simulink model "Symmetry_Inverter"  (Simulink 8.3)
settings: Solver=ode23t  StartTime=0.0  StopTime=tfin  RelTol=1e-4
values from neighbouring files (symbols this model uses):
  amp_feedback_saturation = 400    [Symmetry_ini_COPY.m]
  Bridge_Inductances = 4e-3    (= 0.004)    [Inverter_ini.m]    (also in Symmetry_ini_COPY.m)
  Buffer_Capacitance = 10e-3    (= 0.01)    [Inverter_ini.m]    (also in Symmetry_ini_COPY.m)
  C_Network = [0, 0, 0]    [Symmetry_ini.m]    (also in Symmetry_ini_COPY.m)
  Capacitive_Load_R_RC = [30e-3,  60e-3,  40e-3;                                1e-3, 5e-3, 3e-3]    [Symmetry_ini.m]    (also in Symmetry_ini_COPY.m = [60e-3,  120e-3,  80e-3;                                 1e-)
  Capacitive_Load_S_RC = [30e-3,  60e-3,  40e-3;                                1e-3, 5e-3, 3e-3]    [Symmetry_ini.m]    (also in Symmetry_ini_COPY.m = [60e-3,  120e-3,  80e-3;                                1e-3)
  Capacitive_Load_T_RC = [30e-3,  60e-3,  40e-3;                                1e-3, 5e-3, 3e-3]    [Symmetry_ini.m]    (also in Symmetry_ini_COPY.m = [60e-3,  120e-3,  80e-3;                                 1e-)
  i = str2num(answer{1})/sample    [Test_intersect.m]
  initial_value = [0.00,0.00,0.00,                  0,0,0]    [Symmetry_ini_COPY.m]
  L_Network = [3.185e-3, 3.185e-3, 3.185e-3, 3.185e-3]    [Symmetry_ini.m]    (also in Symmetry_ini_COPY.m)
  L_Source = [3.185e-3, 3.185e-3, 3.185e-3]    [Sketch_controller_model_ini.m]    (also in Symmetry_ini.m; Symmetry_ini_COPY.m)
  Load_R = [50,50,50]    [Symmetry_ini.m]    (also in Symmetry_ini_COPY.m)
  Load_RL = [35.35,   35.35,   35.35;                  0.1125,  0.1125,  0.1125]    [Symmetry_ini.m]    (also in Symmetry_ini_COPY.m = [35.35,   35.35,   35.35;                   0.1125,  0.1125,)
  Load_Wire_Resistance = [0.1,0.2]    [Symmetry_ini.m]    (also in Symmetry_ini_COPY.m)
  P_gain = 0.00001    (= 1e-05)    [Symmetry_ini_COPY.m]
  phase_feedback_saturation = pi    (= 3.14159265359)    [Symmetry_ini_COPY.m]
  Phase_Source = [0,2/3*pi,4/3*pi]    [Sketch_controller_model_ini.m]    (also in Symmetry_REAL_TIME_ini.m = [0,-2/3*pi,-4/3*pi]; Symmetry_ini.m; Symmetry_ini_COPY.m = [0,-2/3*pi,-4/3*pi])
  R_Network = [0.4, 0.4, 0.4, 0.4]    [Symmetry_ini.m]    (also in Symmetry_ini_COPY.m)
  R_Source = [0.4, 0.4, 0.4]    [Sketch_controller_model_ini.m]    (also in Symmetry_ini.m; Symmetry_ini_COPY.m)
  sample = 10e-5    (= 0.0001)    [Inverter_ini.m]    (also in Sketch_controller_model_ini.m; Symmetry_REAL_TIME_ini.m; Symmetry_ini.m; Symmetry_ini_COPY.m)
  Source_Frequency = [50,50,50]    [Sketch_controller_model_ini.m]    (also in Symmetry_ini.m; Symmetry_ini_COPY.m)
  Start_Control = 1    [Symmetry_ini_COPY.m]
  START_Load_R = [0.001,100,100]    [Symmetry_ini_COPY.m]
  START_Load_RC = [100,100,0.001]    [Symmetry_ini_COPY.m]
  START_Load_RL = [100,0.001,100]    [Symmetry_ini_COPY.m]
  step_size = [5,5,5,                  0.36,0.36,0.36]    [Symmetry_ini_COPY.m]
  test_step = [0.5,0.5,0.5,                  0.02,0.02,0.02]    [Symmetry_ini_COPY.m]
  Urms_Source = [230,230,230]    [Sketch_controller_model_ini.m]    (also in Symmetry_REAL_TIME_ini.m; Symmetry_ini.m; Symmetry_ini_COPY.m)
undefined symbols (not defined in the file or in its folder): Ion, Lithium
libraries: powerlib x132, simulink x23, dspsigops x14, commsequence2 x6, dspxfrm3 x3, dsparch4 x2, electricdrivelib x1
(part 2 of 2)

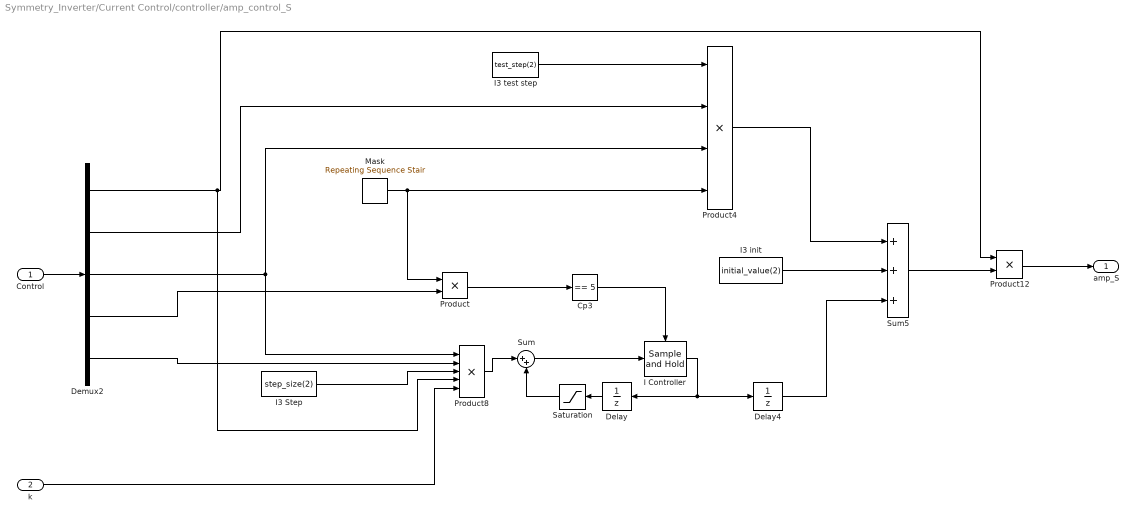
== system Symmetry_Inverter/Current Control/controller/amp_control_S ==
  Control : Inport
  k : Inport  Port=2
  Cp3 : simulink/Logic and Bit Operations/Compare To Constant  relop===  const=5  OutDataTypeStr=uint8  ZeroCross=off
  Delay : UnitDelay  SampleTime=0.001
  Delay4 : UnitDelay  SampleTime=0.02
  Demux2 : Demux  Outputs=5
  I Controller : dspsigops/Sample and Hold  trig=Rising edge  initCond=0  latchinput=off
  I3 Step : Constant  Value=step_size(2)
  "I3 init " : Constant  Value=initial_value(2)
  I3 test step : Constant  Value=test_step(2)
  Mask : simulink/Sources/Repeating Sequence Stair  OutValues=[0 1 0 0 0 0].'  tsamp=mask_sample  OutMin=[]  OutMax=[]  OutDataTypeStr=float('double')  OutputDataTypeScalingMode=Specify via dialog  OutDataType=float('double')  ConRadixGroup=Best Precision: Vector-wise  OutScaling=2^-12
  Product : Product  RndMeth=Zero
  Product12 : Product  RndMeth=Zero
  Product4 : Product  Inputs=4  RndMeth=Zero
  Product8 : Product  Inputs=5  RndMeth=Zero
  Saturation : Saturate  UpperLimit=amp_feedback_saturation  LowerLimit=-amp_feedback_saturation
  Sum : Sum  Inputs=|++
  Sum5 : Sum  Inputs=+++
  amp_S : Outport
  wires:
  Saturation/1 -> Sum/2
  Sum/1 -> I Controller/1
  Product/1 -> Cp3/1
  Product4/1 -> Sum5/1
  I Controller/1 -> Delay/1, Delay4/1
  I3 test step/1 -> Product4/1
  Sum5/1 -> Product12/2
  Mask/1 -> Product4/4, Product/1
  Cp3/1 -> I Controller/Trigger
  I3 Step/1 -> Product8/3
  Demux2/1 -> Product8/4, Product12/1
  Demux2/2 -> Product4/2
  Demux2/3 -> Product8/1, Product4/3
  Demux2/4 -> Product/2
  Demux2/5 -> Product8/2
  Delay4/1 -> Sum5/3
  "I3 init "/1 -> Sum5/2
  Delay/1 -> Saturation/1
  Product8/1 -> Sum/1
  Product12/1 -> amp_S/1
  Control/1 -> Demux2/1
  k/1 -> Product8/5

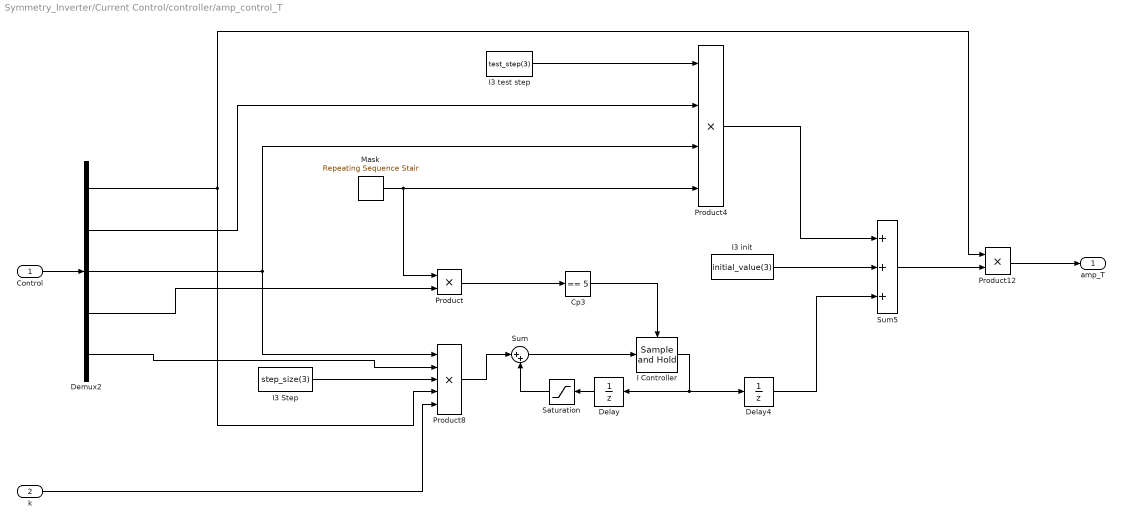
== system Symmetry_Inverter/Current Control/controller/amp_control_T ==
  Control : Inport
  k : Inport  Port=2
  Cp3 : simulink/Logic and Bit Operations/Compare To Constant  relop===  const=5  OutDataTypeStr=uint8  ZeroCross=off
  Delay : UnitDelay  SampleTime=0.001
  Delay4 : UnitDelay  SampleTime=0.02
  Demux2 : Demux  Outputs=5
  I Controller : dspsigops/Sample and Hold  trig=Rising edge  initCond=0  latchinput=off
  I3 Step : Constant  Value=step_size(3)
  "I3 init " : Constant  Value=initial_value(3)
  I3 test step : Constant  Value=test_step(3)
  Mask : simulink/Sources/Repeating Sequence Stair  OutValues=[0 0 1 0 0 0].'  tsamp=mask_sample  OutMin=[]  OutMax=[]  OutDataTypeStr=float('double')  OutputDataTypeScalingMode=Specify via dialog  OutDataType=float('double')  ConRadixGroup=Best Precision: Vector-wise  OutScaling=2^-12
  Product : Product  RndMeth=Zero
  Product12 : Product  RndMeth=Zero
  Product4 : Product  Inputs=4  RndMeth=Zero
  Product8 : Product  Inputs=5  RndMeth=Zero
  Saturation : Saturate  UpperLimit=amp_feedback_saturation  LowerLimit=-amp_feedback_saturation
  Sum : Sum  Inputs=|++
  Sum5 : Sum  Inputs=+++
  amp_T : Outport
  wires:
  Control/1 -> Demux2/1
  Product12/1 -> amp_T/1
  Product8/1 -> Sum/1
  Delay/1 -> Saturation/1
  "I3 init "/1 -> Sum5/2
  Delay4/1 -> Sum5/3
  Demux2/5 -> Product8/2
  Demux2/4 -> Product/2
  Demux2/3 -> Product4/3, Product8/1
  Demux2/2 -> Product4/2
  Demux2/1 -> Product12/1, Product8/4
  I3 Step/1 -> Product8/3
  Cp3/1 -> I Controller/Trigger
  Mask/1 -> Product/1, Product4/4
  Sum5/1 -> Product12/2
  I3 test step/1 -> Product4/1
  I Controller/1 -> Delay4/1, Delay/1
  Product4/1 -> Sum5/1
  Product/1 -> Cp3/1
  Sum/1 -> I Controller/1
  Saturation/1 -> Sum/2
  k/1 -> Product8/5

== system Symmetry_Inverter/Current Control/controller/phase_control_R ==
  Control : Inport
  Cp3 : simulink/Logic and Bit Operations/Compare To Constant  relop===  const=5  OutDataTypeStr=uint8  ZeroCross=off
  Delay : UnitDelay  SampleTime=0.001
  Delay4 : UnitDelay  SampleTime=0.02
  Demux2 : Demux  Outputs=5
  I Controller : dspsigops/Sample and Hold  trig=Rising edge  initCond=0  latchinput=off
  I3 Step : Constant  Value=step_size(4)
  "I3 init " : Constant  Value=initial_value(4)
  I3 test step : Constant  Value=test_step(4)
  Mask : simulink/Sources/Repeating Sequence Stair  OutValues=[0 0 0 1 0 0].'  tsamp=mask_sample  OutMin=[]  OutMax=[]  OutDataTypeStr=float('double')  OutputDataTypeScalingMode=Specify via dialog  OutDataType=float('double')  ConRadixGroup=Best Precision: Vector-wise  OutScaling=2^-12
  Product : Product  RndMeth=Zero
  Product12 : Product  RndMeth=Zero
  Product4 : Product  Inputs=4  RndMeth=Zero
  Product8 : Product  Inputs=4  RndMeth=Zero
  Saturation : Saturate  UpperLimit=phase_feedback_saturation  LowerLimit=-phase_feedback_saturation
  Sum : Sum  Inputs=|++
  Sum5 : Sum  Inputs=+++
  phase_R : Outport
  wires:
  Saturation/1 -> Sum/2
  Sum/1 -> I Controller/1
  Product/1 -> Cp3/1
  Product4/1 -> Sum5/1
  I Controller/1 -> Delay/1, Delay4/1
  I3 test step/1 -> Product4/1
  Sum5/1 -> Product12/2
  Mask/1 -> Product4/4, Product/1
  Cp3/1 -> I Controller/Trigger
  I3 Step/1 -> Product8/3
  Demux2/1 -> Product12/1, Product8/4
  Demux2/2 -> Product4/2
  Demux2/3 -> Product8/1, Product4/3
  Demux2/4 -> Product/2
  Demux2/5 -> Product8/2
  Delay4/1 -> Sum5/3
  "I3 init "/1 -> Sum5/2
  Delay/1 -> Saturation/1
  Product8/1 -> Sum/1
  Product12/1 -> phase_R/1
  Control/1 -> Demux2/1

== system Symmetry_Inverter/Current Control/controller/phase_control_T ==
  Control : Inport
  Cp3 : simulink/Logic and Bit Operations/Compare To Constant  relop===  const=5  OutDataTypeStr=uint8  ZeroCross=off
  Delay : UnitDelay  SampleTime=0.001
  Delay4 : UnitDelay  SampleTime=0.02
  Demux2 : Demux  Outputs=5
  I Controller : dspsigops/Sample and Hold  trig=Rising edge  initCond=0  latchinput=off
  I3 Step : Constant  Value=step_size(6)
  "I3 init " : Constant  Value=initial_value(6)
  I3 test step : Constant  Value=test_step(6)
  Mask : simulink/Sources/Repeating Sequence Stair  OutValues=[0 0 0 0 0 1].'  tsamp=mask_sample  OutMin=[]  OutMax=[]  OutDataTypeStr=float('double')  OutputDataTypeScalingMode=Specify via dialog  OutDataType=float('double')  ConRadixGroup=Best Precision: Vector-wise  OutScaling=2^-12
  Product : Product  RndMeth=Zero
  Product12 : Product  RndMeth=Zero
  Product4 : Product  Inputs=4  RndMeth=Zero
  Product8 : Product  Inputs=4  RndMeth=Zero
  Saturation : Saturate  UpperLimit=phase_feedback_saturation  LowerLimit=-phase_feedback_saturation
  Sum : Sum  Inputs=|++
  Sum5 : Sum  Inputs=+++
  phase_S : Outport
  wires:
  Saturation/1 -> Sum/2
  Sum/1 -> I Controller/1
  Product/1 -> Cp3/1
  Product4/1 -> Sum5/1
  I Controller/1 -> Delay/1, Delay4/1
  I3 test step/1 -> Product4/1
  Sum5/1 -> Product12/2
  Mask/1 -> Product4/4, Product/1
  Cp3/1 -> I Controller/Trigger
  I3 Step/1 -> Product8/3
  Demux2/1 -> Product12/1, Product8/4
  Demux2/2 -> Product4/2
  Demux2/3 -> Product8/1, Product4/3
  Demux2/4 -> Product/2
  Demux2/5 -> Product8/2
  Delay4/1 -> Sum5/3
  "I3 init "/1 -> Sum5/2
  Delay/1 -> Saturation/1
  Product8/1 -> Sum/1
  Product12/1 -> phase_S/1
  Control/1 -> Demux2/1

== system Symmetry_Inverter/Load System/Loads/Capacitive_Loads_RST ==
  Breaker1 : powerlib/Elements/Breaker  InitialState=0  SwitchingTimes="[ 1/60  5/60 ]"  External=on  BreakerResistance=0.01  SnubberResistance=1e7  SnubberCapacitance=inf  Measurements=None  MoreParameters=off  NoBreakLoop=off
  Breaker4 : powerlib/Elements/Breaker  InitialState=0  SwitchingTimes="[ 1/60  5/60 ]"  External=on  BreakerResistance=0.01  SnubberResistance=1e7  SnubberCapacitance=inf  Measurements=None  MoreParameters=off  NoBreakLoop=off
  Breaker6 : powerlib/Elements/Breaker  InitialState=0  SwitchingTimes="[ 1/60  5/60 ]"  External=on  BreakerResistance=0.01  SnubberResistance=1e7  SnubberCapacitance=inf  Measurements=None  MoreParameters=off  NoBreakLoop=off
  Capacitive_Load_R : Subsystem
  Capacitive_Load_S : Subsystem
  Capacitive_Load_T : Subsystem
  Clock : Clock
      settings: Decimation=CLK
  const : Constant
  const1 : Constant  Value=0
  on/off : Switch  Criteria=u2 > Threshold  Threshold=START_Load_RC(1)
  on/off1 : Switch  Criteria=u2 > Threshold  Threshold=START_Load_RC(2)
  on/off2 : Switch  Criteria=u2 > Threshold  Threshold=START_Load_RC(3)
  R : PMIOPort  Port=1  Side=Right
  S : PMIOPort  Port=2  Side=Right
  T : PMIOPort  Port=3  Side=Right
  N : PMIOPort  Port=4  Side=Left
  wires:
  const/1 -> on/off2/1, on/off1/1, on/off/1
  const1/1 -> on/off2/3, on/off1/3, on/off/3
  Clock/1 -> on/off2/2, on/off1/2, on/off/2
  on/off/1 -> Breaker4/1
  on/off1/1 -> Breaker1/1
  on/off2/1 -> Breaker6/1
  connections:
  R/RConn1 -- Breaker4/LConn1
  S/RConn1 -- Breaker1/LConn1
  T/RConn1 -- Breaker6/LConn1
  Capacitive_Load_R/LConn1 -- Breaker4/RConn1
  Capacitive_Load_S/LConn1 -- Breaker1/RConn1
  Capacitive_Load_T/LConn1 -- Breaker6/RConn1
  Capacitive_Load_R/LConn2 -- Capacitive_Load_S/LConn2 -- Capacitive_Load_T/LConn2 -- N/RConn1

== system Symmetry_Inverter/Load System/Loads/Inductive_Loads_RST ==
  Breaker1 : powerlib/Elements/Breaker  InitialState=0  SwitchingTimes="[ 1/60  5/60 ]"  External=on  BreakerResistance=0.01  SnubberResistance=1e7  SnubberCapacitance=inf  Measurements=None  MoreParameters=off  NoBreakLoop=off
  Breaker13 : powerlib/Elements/Breaker  InitialState=0  SwitchingTimes="[ 1/60  5/60 ]"  External=on  BreakerResistance=0.01  SnubberResistance=1e7  SnubberCapacitance=inf  Measurements=None  MoreParameters=off  NoBreakLoop=off
  Breaker2 : powerlib/Elements/Breaker  InitialState=0  SwitchingTimes="[ 1/60  5/60 ]"  External=on  BreakerResistance=0.01  SnubberResistance=1e7  SnubberCapacitance=inf  Measurements=None  MoreParameters=off  NoBreakLoop=off
  Clock : Clock
      settings: Decimation=CLK
  RL_load : powerlib/Elements/Series RLC Branch  LConnTagsString=__new0  RConnTagsString=__new0  BranchType=RL  Resistance=Load_RL(1,1)  Inductance=Load_RL(2,1)  SetiL0=off  InitialCurrent=0  Capacitance=1.0  Setx0=off  InitialVoltage=0  Measurements=None
  RL_load1 : powerlib/Elements/Series RLC Branch  LConnTagsString=__new0  RConnTagsString=__new0  BranchType=RL  Resistance=Load_RL(1,2)  Inductance=Load_RL(2,2)  SetiL0=off  InitialCurrent=0  Capacitance=1.0  Setx0=off  InitialVoltage=0  Measurements=None
  RL_load2 : powerlib/Elements/Series RLC Branch  LConnTagsString=__new0  RConnTagsString=__new0  BranchType=RL  Resistance=Load_RL(1,3)  Inductance=Load_RL(2,3)  SetiL0=off  InitialCurrent=0  Capacitance=1.0  Setx0=off  InitialVoltage=0  Measurements=None
  const : Constant
  const1 : Constant  Value=0
  on/off : Switch  Criteria=u2 > Threshold  Threshold=START_Load_RL(1)
  on/off1 : Switch  Criteria=u2 > Threshold  Threshold=START_Load_RL(2)
  on/off2 : Switch  Criteria=u2 > Threshold  Threshold=START_Load_RL(3)
  R : PMIOPort  Port=1  Side=Left
  S : PMIOPort  Port=2  Side=Left
  T : PMIOPort  Port=3  Side=Left
  N : PMIOPort  Port=4  Side=Right
  wires:
  const/1 -> on/off2/1, on/off1/1, on/off/1
  const1/1 -> on/off2/3, on/off1/3, on/off/3
  Clock/1 -> on/off2/2, on/off1/2, on/off/2
  on/off/1 -> Breaker13/1
  on/off1/1 -> Breaker1/1
  on/off2/1 -> Breaker2/1
  connections:
  RL_load/RConn1 -- RL_load1/RConn1 -- RL_load2/RConn1 -- N/RConn1
  R/RConn1 -- Breaker13/LConn1
  Breaker1/LConn1 -- S/RConn1
  Breaker2/LConn1 -- T/RConn1
  Breaker13/RConn1 -- RL_load/LConn1
  RL_load1/LConn1 -- Breaker1/RConn1
  RL_load2/LConn1 -- Breaker2/RConn1

== system Symmetry_Inverter/Load System/Loads/Ohmic_Loads_RST ==
  Breaker1 : powerlib/Elements/Breaker  InitialState=0  SwitchingTimes="[ 1/60  5/60 ]"  External=on  BreakerResistance=0.01  SnubberResistance=1e7  SnubberCapacitance=inf  Measurements=None  MoreParameters=off  NoBreakLoop=off
  Breaker13 : powerlib/Elements/Breaker  InitialState=0  SwitchingTimes="[ 1/60  5/60 ]"  External=on  BreakerResistance=0.01  SnubberResistance=1e7  SnubberCapacitance=inf  Measurements=None  MoreParameters=off  NoBreakLoop=off
  Breaker2 : powerlib/Elements/Breaker  InitialState=0  SwitchingTimes="[ 1/60  5/60 ]"  External=on  BreakerResistance=0.01  SnubberResistance=1e7  SnubberCapacitance=inf  Measurements=None  MoreParameters=off  NoBreakLoop=off
  Clock : Clock
      settings: Decimation=CLK
  R_load : powerlib/Elements/Series RLC Branch  LConnTagsString=__new0  RConnTagsString=__new0  BranchType=R  Resistance=Load_R(1)  Inductance=0.003185  SetiL0=off  InitialCurrent=0  Capacitance=1.0  Setx0=off  InitialVoltage=0  Measurements=None
  R_load1 : powerlib/Elements/Series RLC Branch  LConnTagsString=__new0  RConnTagsString=__new0  BranchType=R  Resistance=Load_R(2)  Inductance=0.003185  SetiL0=off  InitialCurrent=0  Capacitance=1.0  Setx0=off  InitialVoltage=0  Measurements=None
  R_load2 : powerlib/Elements/Series RLC Branch  LConnTagsString=__new0  RConnTagsString=__new0  BranchType=R  Resistance=Load_R(3)  Inductance=0.003185  SetiL0=off  InitialCurrent=0  Capacitance=1.0  Setx0=off  InitialVoltage=0  Measurements=None
  const : Constant
  const1 : Constant  Value=0
  on/off : Switch  Criteria=u2 > Threshold  Threshold=START_Load_R(1)
  on/off1 : Switch  Criteria=u2 > Threshold  Threshold=START_Load_R(2)
  on/off2 : Switch  Criteria=u2 > Threshold  Threshold=START_Load_R(3)
  R : PMIOPort  Port=1  Side=Left
  S : PMIOPort  Port=2  Side=Left
  T : PMIOPort  Port=3  Side=Left
  N : PMIOPort  Port=4  Side=Right
  wires:
  const/1 -> on/off2/1, on/off1/1, on/off/1
  const1/1 -> on/off2/3, on/off1/3, on/off/3
  Clock/1 -> on/off2/2, on/off1/2, on/off/2
  on/off/1 -> Breaker13/1
  on/off1/1 -> Breaker1/1
  on/off2/1 -> Breaker2/1
  connections:
  R_load/RConn1 -- R_load1/RConn1 -- R_load2/RConn1 -- N/RConn1
  Breaker13/LConn1 -- R/RConn1
  Breaker13/RConn1 -- R_load/LConn1
  Breaker1/LConn1 -- S/RConn1
  R_load1/LConn1 -- Breaker1/RConn1
  Breaker2/LConn1 -- T/RConn1
  R_load2/LConn1 -- Breaker2/RConn1

== system Symmetry_Inverter/Current Control/Grid Synchronized Inverter/Inverter_Bridge_R/Bridge Controller R ==
  In1 : Inport
  I out contr 1 : Relay  OnSwitchValue=0.01  OffSwitchValue=-0.01  OnOutputValue=10  ZeroCross=off  SampleTime=1e-6
  I out contr 2 : Relay  OnSwitchValue=0.01  OffSwitchValue=-0.01  OnOutputValue=0  OffOutputValue=10  ZeroCross=off  SampleTime=1e-6
  Out1 : Outport
  Out2 : Outport  Port=2
  wires:
  In1/1 -> I out contr 1/1, I out contr 2/1
  I out contr 1/1 -> Out1/1
  I out contr 2/1 -> Out2/1

== system Symmetry_Inverter/Current Control/Grid Synchronized Inverter/Inverter_Bridge_R1/Bridge Controller R ==
  In1 : Inport
  I out contr 1 : Relay  OnSwitchValue=0.01  OffSwitchValue=-0.01  OnOutputValue=10  ZeroCross=off  SampleTime=1e-6
  I out contr 2 : Relay  OnSwitchValue=0.01  OffSwitchValue=-0.01  OnOutputValue=0  OffOutputValue=10  ZeroCross=off  SampleTime=1e-6
  Out1 : Outport
  Out2 : Outport  Port=2
  wires:
  I out contr 2/1 -> Out2/1
  I out contr 1/1 -> Out1/1
  In1/1 -> I out contr 2/1, I out contr 1/1

== system Symmetry_Inverter/Current Control/Grid Synchronized Inverter/Inverter_Bridge_R2/Bridge Controller R ==
  In1 : Inport
  I out contr 1 : Relay  OnSwitchValue=0.01  OffSwitchValue=-0.01  OnOutputValue=10  ZeroCross=off  SampleTime=1e-6
  I out contr 2 : Relay  OnSwitchValue=0.01  OffSwitchValue=-0.01  OnOutputValue=0  OffOutputValue=10  ZeroCross=off  SampleTime=1e-6
  Out1 : Outport
  Out2 : Outport  Port=2
  wires:
  In1/1 -> I out contr 1/1, I out contr 2/1
  I out contr 1/1 -> Out1/1
  I out contr 2/1 -> Out2/1

== system Symmetry_Inverter/Load System/Loads/Capacitive_Loads_RST/Capacitive_Load_R ==
  Capacitive_Load_R_1 : Subsystem
  Capacitive_Load_R_2 : Subsystem
  Capacitive_Load_R_3 : Subsystem
  AC : PMIOPort  Port=1  Side=Left
  N : PMIOPort  Port=2  Side=Left
  connections:
  N/RConn1 -- Capacitive_Load_R_3/LConn2 -- Capacitive_Load_R_2/LConn2 -- Capacitive_Load_R_1/RConn2
  Capacitive_Load_R_2/LConn1 -- Capacitive_Load_R_1/RConn1 -- Capacitive_Load_R_3/LConn1 -- AC/RConn1

== system Symmetry_Inverter/Load System/Loads/Capacitive_Loads_RST/Capacitive_Load_S ==
  Capacitive_Load_S_1 : Subsystem
  Capacitive_Load_S_2 : Subsystem
  Capacitive_Load_S_3 : Subsystem
  AC : PMIOPort  Port=1  Side=Left
  N : PMIOPort  Port=2  Side=Left
  connections:
  AC/RConn1 -- Capacitive_Load_S_3/LConn1 -- Capacitive_Load_S_1/RConn1 -- Capacitive_Load_S_2/LConn1
  Capacitive_Load_S_1/RConn2 -- Capacitive_Load_S_2/LConn2 -- Capacitive_Load_S_3/LConn2 -- N/RConn1

== system Symmetry_Inverter/Load System/Loads/Capacitive_Loads_RST/Capacitive_Load_T ==
  Capacitive_Load_R_1 : Subsystem
  Capacitive_Load_R_2 : Subsystem
  Capacitive_Load_R_3 : Subsystem
  AC : PMIOPort  Port=1  Side=Left
  N : PMIOPort  Port=2  Side=Left
  connections:
  N/RConn1 -- Capacitive_Load_R_3/LConn2 -- Capacitive_Load_R_2/LConn2 -- Capacitive_Load_R_1/RConn2
  Capacitive_Load_R_2/LConn1 -- Capacitive_Load_R_1/RConn1 -- Capacitive_Load_R_3/LConn1 -- AC/RConn1

== system Symmetry_Inverter/Load System/Loads/Capacitive_Loads_RST/Capacitive_Load_R/Capacitive_Load_R_1 ==
  Breaker5 : powerlib/Elements/Breaker  InitialState=0  SwitchingTimes="[ 1/60  5/60 ]"  External=on  BreakerResistance=0.01  SnubberResistance=1e7  SnubberCapacitance=inf  Measurements=None  MoreParameters=off  NoBreakLoop=off
  Constant : Constant
  Series RLC Branch : powerlib/Elements/Series RLC Branch  LConnTagsString=__new0  RConnTagsString=__new0  BranchType=RC  Resistance=Capacitive_Load_R_RC(1,1)  Inductance=1e-3  SetiL0=off  InitialCurrent=0  Capacitance=Capacitive_Load_R_RC(2,1)  Setx0=off  InitialVoltage=0  Measurements=None
  Universal Bridge : powerlib/Power Electronics/Universal Bridge  Arms=2  SnubberResistance=1e5  SnubberCapacitance=inf  Device=Diodes  Ron=1e-3  Lon=0  ForwardVoltages="[  0  0  ]"  ForwardVoltage=0.8  GTOparameters=[ 10e-6 , 20e-6 ]  IGBTparameters=[ 1e-6 , 2e-6 ]  Measurements=None  Measurements_2=None  converterType=Rectifier
  AC : PMIOPort  Port=1  Side=Right
  N : PMIOPort  Port=2  Side=Right
  wires:
  Constant/1 -> Breaker5/1
  connections:
  Universal Bridge/LConn2 -- N/RConn1
  Breaker5/RConn1 -- Universal Bridge/LConn1
  AC/RConn1 -- Breaker5/LConn1
  Universal Bridge/RConn1 -- Series RLC Branch/LConn1
  Universal Bridge/RConn2 -- Series RLC Branch/RConn1

== system Symmetry_Inverter/Load System/Loads/Capacitive_Loads_RST/Capacitive_Load_R/Capacitive_Load_R_2 ==
  Breaker2 : powerlib/Elements/Breaker  InitialState=0  SwitchingTimes="[ 1/60  5/60 ]"  External=on  BreakerResistance=0.01  SnubberResistance=1e7  SnubberCapacitance=inf  Measurements=None  MoreParameters=off  NoBreakLoop=off
  Constant : Constant
  Series RLC Branch : powerlib/Elements/Series RLC Branch  LConnTagsString=__new0  RConnTagsString=__new0  BranchType=RC  Resistance=Capacitive_Load_R_RC(1,2)  Inductance=1e-3  SetiL0=off  InitialCurrent=0  Capacitance=Capacitive_Load_R_RC(2,2)  Setx0=off  InitialVoltage=0  Measurements=None
  Universal Bridge1 : powerlib/Power Electronics/Universal Bridge  Arms=2  SnubberResistance=1e5  SnubberCapacitance=inf  Device=Diodes  Ron=1e-3  Lon=0  ForwardVoltages="[  0  0  ]"  ForwardVoltage=0.8  GTOparameters=[ 10e-6 , 20e-6 ]  IGBTparameters=[ 1e-6 , 2e-6 ]  Measurements=None  Measurements_2=None  converterType=Rectifier
  AC : PMIOPort  Port=1  Side=Left
  N : PMIOPort  Port=2  Side=Left
  wires:
  Constant/1 -> Breaker2/1
  connections:
  Universal Bridge1/LConn2 -- N/RConn1
  Breaker2/RConn1 -- Universal Bridge1/LConn1
  AC/RConn1 -- Breaker2/LConn1
  Series RLC Branch/LConn1 -- Universal Bridge1/RConn1
  Series RLC Branch/RConn1 -- Universal Bridge1/RConn2

== system Symmetry_Inverter/Load System/Loads/Capacitive_Loads_RST/Capacitive_Load_R/Capacitive_Load_R_3 ==
  Breaker3 : powerlib/Elements/Breaker  InitialState=0  SwitchingTimes="[ 1/60  5/60 ]"  External=on  BreakerResistance=0.01  SnubberResistance=1e7  SnubberCapacitance=inf  Measurements=None  MoreParameters=off  NoBreakLoop=off
  Constant : Constant
  Series RLC Branch : powerlib/Elements/Series RLC Branch  LConnTagsString=__new0  RConnTagsString=__new0  BranchType=RC  Resistance=Capacitive_Load_R_RC(1,3)  Inductance=1e-3  SetiL0=off  InitialCurrent=0  Capacitance=Capacitive_Load_R_RC(2,3)  Setx0=off  InitialVoltage=0  Measurements=None
  Universal Bridge2 : powerlib/Power Electronics/Universal Bridge  Arms=2  SnubberResistance=1e5  SnubberCapacitance=inf  Device=Diodes  Ron=1e-3  Lon=0  ForwardVoltages="[  0  0  ]"  ForwardVoltage=0.8  GTOparameters=[ 10e-6 , 20e-6 ]  IGBTparameters=[ 1e-6 , 2e-6 ]  Measurements=None  Measurements_2=None  converterType=Rectifier
  AC : PMIOPort  Port=1  Side=Left
  "N " : PMIOPort  Port=2  Side=Left
  wires:
  Constant/1 -> Breaker3/1
  connections:
  Breaker3/RConn1 -- Universal Bridge2/LConn1
  Universal Bridge2/LConn2 -- "N "/RConn1
  AC/RConn1 -- Breaker3/LConn1
  Series RLC Branch/LConn1 -- Universal Bridge2/RConn1
  Series RLC Branch/RConn1 -- Universal Bridge2/RConn2

== system Symmetry_Inverter/Load System/Loads/Capacitive_Loads_RST/Capacitive_Load_S/Capacitive_Load_S_1 ==
  Breaker5 : powerlib/Elements/Breaker  InitialState=0  SwitchingTimes="[ 1/60  5/60 ]"  External=on  BreakerResistance=0.01  SnubberResistance=1e7  SnubberCapacitance=inf  Measurements=None  MoreParameters=off  NoBreakLoop=off
  Constant : Constant
  Series RLC Branch : powerlib/Elements/Series RLC Branch  LConnTagsString=__new0  RConnTagsString=__new0  BranchType=RC  Resistance=Capacitive_Load_S_RC(1,1)  Inductance=1e-3  SetiL0=off  InitialCurrent=0  Capacitance=Capacitive_Load_S_RC(2,1)  Setx0=off  InitialVoltage=0  Measurements=None
  Universal Bridge : powerlib/Power Electronics/Universal Bridge  Arms=2  SnubberResistance=1e5  SnubberCapacitance=inf  Device=Diodes  Ron=1e-3  Lon=0  ForwardVoltages="[  0  0  ]"  ForwardVoltage=0.8  GTOparameters=[ 10e-6 , 20e-6 ]  IGBTparameters=[ 1e-6 , 2e-6 ]  Measurements=None  Measurements_2=None  converterType=Rectifier
  AC : PMIOPort  Port=1  Side=Right
  N : PMIOPort  Port=2  Side=Right
  wires:
  Constant/1 -> Breaker5/1
  connections:
  AC/RConn1 -- Breaker5/LConn1
  Breaker5/RConn1 -- Universal Bridge/LConn1
  Universal Bridge/LConn2 -- N/RConn1
  Series RLC Branch/LConn1 -- Universal Bridge/RConn1
  Series RLC Branch/RConn1 -- Universal Bridge/RConn2

== system Symmetry_Inverter/Load System/Loads/Capacitive_Loads_RST/Capacitive_Load_S/Capacitive_Load_S_2 ==
  Breaker2 : powerlib/Elements/Breaker  InitialState=0  SwitchingTimes="[ 1/60  5/60 ]"  External=on  BreakerResistance=0.01  SnubberResistance=1e7  SnubberCapacitance=inf  Measurements=None  MoreParameters=off  NoBreakLoop=off
  Constant : Constant
  Series RLC Branch : powerlib/Elements/Series RLC Branch  LConnTagsString=__new0  RConnTagsString=__new0  BranchType=RC  Resistance=Capacitive_Load_S_RC(1,2)  Inductance=1e-3  SetiL0=off  InitialCurrent=0  Capacitance=Capacitive_Load_S_RC(2,2)  Setx0=off  InitialVoltage=0  Measurements=None
  Universal Bridge1 : powerlib/Power Electronics/Universal Bridge  Arms=2  SnubberResistance=1e5  SnubberCapacitance=inf  Device=Diodes  Ron=1e-3  Lon=0  ForwardVoltages="[  0  0  ]"  ForwardVoltage=0.8  GTOparameters=[ 10e-6 , 20e-6 ]  IGBTparameters=[ 1e-6 , 2e-6 ]  Measurements=None  Measurements_2=None  converterType=Rectifier
  AC : PMIOPort  Port=1  Side=Left
  N : PMIOPort  Port=2  Side=Left
  wires:
  Constant/1 -> Breaker2/1
  connections:
  AC/RConn1 -- Breaker2/LConn1
  Breaker2/RConn1 -- Universal Bridge1/LConn1
  Universal Bridge1/LConn2 -- N/RConn1
  Series RLC Branch/LConn1 -- Universal Bridge1/RConn1
  Series RLC Branch/RConn1 -- Universal Bridge1/RConn2

== system Symmetry_Inverter/Load System/Loads/Capacitive_Loads_RST/Capacitive_Load_S/Capacitive_Load_S_3 ==
  Breaker3 : powerlib/Elements/Breaker  InitialState=0  SwitchingTimes="[ 1/60  5/60 ]"  External=on  BreakerResistance=0.01  SnubberResistance=1e7  SnubberCapacitance=inf  Measurements=None  MoreParameters=off  NoBreakLoop=off
  Constant : Constant
  Series RLC Branch : powerlib/Elements/Series RLC Branch  LConnTagsString=__new0  RConnTagsString=__new0  BranchType=RC  Resistance=Capacitive_Load_S_RC(1,3)  Inductance=1e-3  SetiL0=off  InitialCurrent=0  Capacitance=Capacitive_Load_S_RC(2,3)  Setx0=off  InitialVoltage=0  Measurements=None
  Universal Bridge2 : powerlib/Power Electronics/Universal Bridge  Arms=2  SnubberResistance=1e5  SnubberCapacitance=inf  Device=Diodes  Ron=1e-3  Lon=0  ForwardVoltages="[  0  0  ]"  ForwardVoltage=0.8  GTOparameters=[ 10e-6 , 20e-6 ]  IGBTparameters=[ 1e-6 , 2e-6 ]  Measurements=None  Measurements_2=None  converterType=Rectifier
  AC : PMIOPort  Port=1  Side=Left
  "N " : PMIOPort  Port=2  Side=Left
  wires:
  Constant/1 -> Breaker3/1
  connections:
  AC/RConn1 -- Breaker3/LConn1
  Universal Bridge2/LConn2 -- "N "/RConn1
  Breaker3/RConn1 -- Universal Bridge2/LConn1
  Series RLC Branch/LConn1 -- Universal Bridge2/RConn1
  Series RLC Branch/RConn1 -- Universal Bridge2/RConn2

== system Symmetry_Inverter/Load System/Loads/Capacitive_Loads_RST/Capacitive_Load_T/Capacitive_Load_R_1 ==
  Breaker5 : powerlib/Elements/Breaker  InitialState=0  SwitchingTimes="[ 1/60  5/60 ]"  External=on  BreakerResistance=0.01  SnubberResistance=1e7  SnubberCapacitance=inf  Measurements=None  MoreParameters=off  NoBreakLoop=off
  Constant : Constant
  Series RLC Branch : powerlib/Elements/Series RLC Branch  LConnTagsString=__new0  RConnTagsString=__new0  BranchType=RC  Resistance=Capacitive_Load_T_RC(1,1)  Inductance=1e-3  SetiL0=off  InitialCurrent=0  Capacitance=Capacitive_Load_T_RC(2,1)  Setx0=off  InitialVoltage=0  Measurements=None
  Universal Bridge : powerlib/Power Electronics/Universal Bridge  Arms=2  SnubberResistance=1e5  SnubberCapacitance=inf  Device=Diodes  Ron=1e-3  Lon=0  ForwardVoltages="[  0  0  ]"  ForwardVoltage=0.8  GTOparameters=[ 10e-6 , 20e-6 ]  IGBTparameters=[ 1e-6 , 2e-6 ]  Measurements=None  Measurements_2=None  converterType=Rectifier
  AC : PMIOPort  Port=1  Side=Right
  N : PMIOPort  Port=2  Side=Right
  wires:
  Constant/1 -> Breaker5/1
  connections:
  Universal Bridge/LConn2 -- N/RConn1
  Breaker5/RConn1 -- Universal Bridge/LConn1
  AC/RConn1 -- Breaker5/LConn1
  Series RLC Branch/RConn1 -- Universal Bridge/RConn2
  Series RLC Branch/LConn1 -- Universal Bridge/RConn1

== system Symmetry_Inverter/Load System/Loads/Capacitive_Loads_RST/Capacitive_Load_T/Capacitive_Load_R_2 ==
  Breaker2 : powerlib/Elements/Breaker  InitialState=0  SwitchingTimes="[ 1/60  5/60 ]"  External=on  BreakerResistance=0.01  SnubberResistance=1e7  SnubberCapacitance=inf  Measurements=None  MoreParameters=off  NoBreakLoop=off
  Constant : Constant
  Series RLC Branch : powerlib/Elements/Series RLC Branch  LConnTagsString=__new0  RConnTagsString=__new0  BranchType=RC  Resistance=Capacitive_Load_T_RC(1,2)  Inductance=1e-3  SetiL0=off  InitialCurrent=0  Capacitance=Capacitive_Load_T_RC(2,2)  Setx0=off  InitialVoltage=0  Measurements=None
  Universal Bridge1 : powerlib/Power Electronics/Universal Bridge  Arms=2  SnubberResistance=1e5  SnubberCapacitance=inf  Device=Diodes  Ron=1e-3  Lon=0  ForwardVoltages="[  0  0  ]"  ForwardVoltage=0.8  GTOparameters=[ 10e-6 , 20e-6 ]  IGBTparameters=[ 1e-6 , 2e-6 ]  Measurements=None  Measurements_2=None  converterType=Rectifier
  AC : PMIOPort  Port=1  Side=Left
  N : PMIOPort  Port=2  Side=Left
  wires:
  Constant/1 -> Breaker2/1
  connections:
  Universal Bridge1/LConn2 -- N/RConn1
  Breaker2/RConn1 -- Universal Bridge1/LConn1
  AC/RConn1 -- Breaker2/LConn1
  Series RLC Branch/RConn1 -- Universal Bridge1/RConn2
  Series RLC Branch/LConn1 -- Universal Bridge1/RConn1

== system Symmetry_Inverter/Load System/Loads/Capacitive_Loads_RST/Capacitive_Load_T/Capacitive_Load_R_3 ==
  Breaker3 : powerlib/Elements/Breaker  InitialState=0  SwitchingTimes="[ 1/60  5/60 ]"  External=on  BreakerResistance=0.01  SnubberResistance=1e7  SnubberCapacitance=inf  Measurements=None  MoreParameters=off  NoBreakLoop=off
  Constant : Constant
  Series RLC Branch : powerlib/Elements/Series RLC Branch  LConnTagsString=__new0  RConnTagsString=__new0  BranchType=RC  Resistance=Capacitive_Load_T_RC(1,3)  Inductance=1e-3  SetiL0=off  InitialCurrent=0  Capacitance=Capacitive_Load_T_RC(2,3)  Setx0=off  InitialVoltage=0  Measurements=None
  Universal Bridge2 : powerlib/Power Electronics/Universal Bridge  Arms=2  SnubberResistance=1e5  SnubberCapacitance=inf  Device=Diodes  Ron=1e-3  Lon=0  ForwardVoltages="[  0  0  ]"  ForwardVoltage=0.8  GTOparameters=[ 10e-6 , 20e-6 ]  IGBTparameters=[ 1e-6 , 2e-6 ]  Measurements=None  Measurements_2=None  converterType=Rectifier
  AC : PMIOPort  Port=1  Side=Left
  "N " : PMIOPort  Port=2  Side=Left
  wires:
  Constant/1 -> Breaker3/1
  connections:
  Breaker3/RConn1 -- Universal Bridge2/LConn1
  Universal Bridge2/LConn2 -- "N "/RConn1
  AC/RConn1 -- Breaker3/LConn1
  Series RLC Branch/RConn1 -- Universal Bridge2/RConn2
  Series RLC Branch/LConn1 -- Universal Bridge2/RConn1

== matlab function Calculate_Norms/Mearusement_calc/vectorial norm ==
  data: amplitude_R input double; VEC_norm output double; amplitude_S input double; amplitude_T input double; phase_R input double; phase_S input double; phase_T input double
function VEC_norm = fcn(amplitude_R,amplitude_S,amplitude_T,phase_R,phase_S,phase_T)
%#codegen

  
   N=complex(0);
   V_real=complex([0,0,0]');
   V_012=complex([0,0,0]');
   V_real(1)=amplitude_R.*exp(1i*phase_R);
   V_real(2)=amplitude_S.*exp(1i*phase_S);
   V_real(3)=amplitude_T.*exp(1i*phase_T); 

   R_error=230*exp(1j*-0/360*2*pi)  -V_real(1);
   S_error=230*exp(1j*-120/360*2*pi)-V_real(2);
   T_error=230*exp(1j*-240/360*2*pi)-V_real(3);
   VEC_norm=abs(R_error*S_error)+abs(R_error*T_error)+abs(S_error*T_error);
   %N=R_error*S_error+R_error*T_error+S_error*T_error;
   %VEC_norm=abs(N);

== matlab function Current Control/controller/MATLAB Function ==
  data: amp input double; CC output double; phase input double; t input double
function CC = fcn(amp,phase,t)
%#codegen


CC_mtx=[amp(1),50,phase(1),0;...
        amp(2),50,phase(2),0;...
        amp(3),50,phase(3),0];
% T=1;
% CC=[(CC_mtx(1,1)*sin(2*pi*CC_mtx(1,2)*t+CC_mtx(1,3))+CC_mtx(1,4)).*(1-exp(-t/T)),...
%     (CC_mtx(2,1)*sin(2*pi*CC_mtx(2,2)*t+CC_mtx(2,3))+CC_mtx(2,4)).*(1-exp(-t/T)),...
%     (CC_mtx(3,1)*sin(2*pi*CC_mtx(3,2)*t+CC_mtx(3,3))+CC_mtx(3,4)).*(1-exp(-t/T))]';

CC=[(CC_mtx(1,1)*sin(2*pi*CC_mtx(1,2)*t+CC_mtx(1,3))+CC_mtx(1,4)),...
    (CC_mtx(2,1)*sin(2*pi*CC_mtx(2,2)*t+CC_mtx(2,3))+CC_mtx(2,4)),...
    (CC_mtx(3,1)*sin(2*pi*CC_mtx(3,2)*t+CC_mtx(3,3))+CC_mtx(3,4))]';
